simulink model "untitledSM1"  (R2019b)
settings: Solver=VariableStepAuto  StartTime=0.0  StopTime=10.0  RelTol=1e-3
settings Model: Creator=edmon  LastModifiedBy=edmon

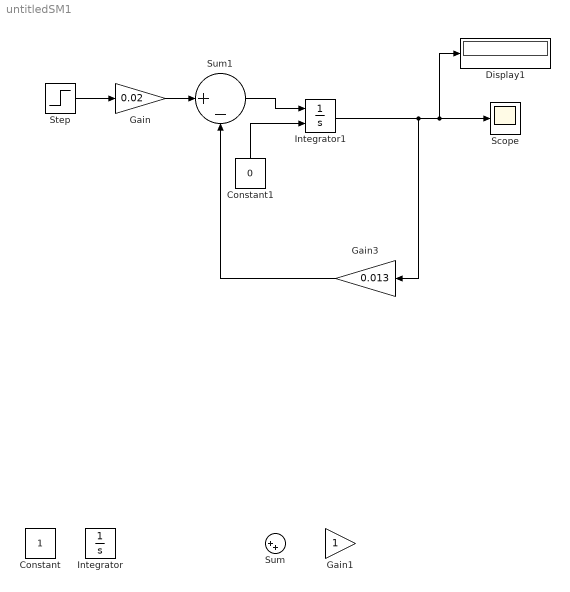
== system untitledSM1 ==
  Constant : Constant
  Constant1 : Constant  Value=0
  Display1 : Display
  Gain : Gain  Gain=0.02
  Gain1 : Gain
  Gain3 : Gain  Gain=0.013
  Integrator : Integrator
  Integrator1 : Integrator  InitialConditionSource=external
  Scope : Scope
  Step : Step  SampleTime=0
  Sum : Sum  Inputs=|++
  Sum1 : Sum  Inputs=|+-
  wires:
  Gain/1 -> Sum1/1
  Gain3/1 -> Sum1/2
  Integrator1/1 -> Gain3/1, Display1/1, Scope/1
  Step/1 -> Gain/1
  Constant1/1 -> Integrator1/2
  Sum1/1 -> Integrator1/1
